simulink model "sf_mask_basic"  (R2017b)
settings: Solver=VariableStepDiscrete  StartTime=0.0  StopTime=300.0  MaxStep=2.0  RelTol=1e-3  EnableMultiTasking=on
libraries: sf_mask_lib x1
settings Model: Creator=The MathWorks, Inc.  LastModifiedBy=The MathWorks, Inc.
settings DataIOCC: LimitDataPoints=on  SaveFormat=Array
settings OptimizationCC: ExpressionDepthLimit=2147483647  LifeSpan=inf
settings DebuggingCC: UnderspecifiedInitializationDetection=Classic  MergeDetectMultiDrivingBlocksExec=none  SolverPrmCheckMsg=warning  StateNameClashWarn=warning  SFUnexpectedBacktrackingDiag=warning  SFNoUnconditionalDefaultTransitionDiag=warning  SFExecutionAtInitializationDiag=none
settings HardwareCC: ProdBitPerPointer=32  ProdBitPerSizeT=32  ProdBitPerPtrDiffT=32  ProdLargestAtomicFloat=None  ProdIntDivRoundTo=Undefined  ProdEndianess=Unspecified  ProdWordSize=32  ProdHWDeviceType=32-bit Generic
settings ModelReferenceCC: PropagateSignalLabelsOutOfModel=off
settings CodeAppCC: StateflowObjectComments=on
settings GRTTargetCC: TargetLangStandard=C89/C90 (ANSI)  GeneratePreprocessorConditionals=Disable all
settings ConfigComp: CovMetricSettings=dw  CovHtmlReporting=on  CovSaveCumulativeToWorkspaceVar=on  CovSaveSingleToWorkspaceVar=on  CovExternalEMLEnable=off

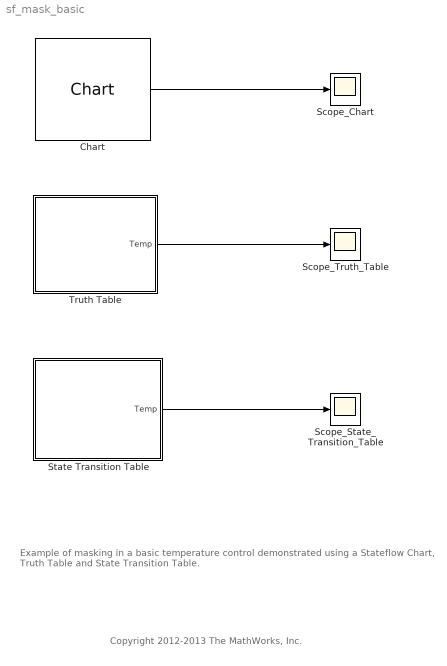
== system sf_mask_basic ==
  note: Copyright 2012-2013 The MathWorks, Inc.
  note: Example of masking in a basic temperature control demonstrated using a
      |  Stateflow Chart, Truth Table and State Transition Table.
  Chart : sf_mask_lib/Chart  AmbTemp=85  DesiredTemp=70  btuSetting=20000 BTUs
      settings: SourceProductName=Stateflow  SourceProductBaseCode=SF
  Scope_Chart : Scope
  Scope_State_Transition_Table : Scope
  Scope_Truth_Table : Scope
  State Transition Table : State Transition Table  TreatAsAtomicUnit=on  mask{AmbTemp=85, DesiredTemp=70, btuSetting=20000 BTU}
      mask prompts: AmbTemp "Ambient Temperature"; DesiredTemp "Desired Temperature"; btuSetting "AC Power"
      mask init:
      | if btuSetting == 1
      |     btuValue = 10000;
      | elseif btuSetting == 2
      |     btuValue = 20000;
      | end
  Truth Table : Truth Table  TreatAsAtomicUnit=on  mask{AmbTemp=85, DesiredTemp=70, btuSetting=20000 BTU}
      mask prompts: AmbTemp "Ambient Temperature"; DesiredTemp "Desired Temperature"; btuSetting "AC Power"
      mask init:
      | if btuSetting == 1
      |     btuValue = 10000;
      | elseif btuSetting == 2
      |     btuValue = 20000;
      | end
  wires:
  Chart/1 -> Scope_Chart/1
  Truth Table/1(Temp) -> Scope_Truth_Table/1
  State Transition Table/1(Temp) -> Scope_State_Transition_Table/1

== matlab function sf_mask_basic/Truth Table ==
  data: Temp output; AmbTemp parameter double; DesiredTemp parameter double; TempStore local double =AmbTemp; btuValue parameter double
function Temp = fcn(AmbTemp, DesiredTemp, btuValue)

INIT();

aVarTruthTableCondition_1 = false;


% Temperature is Less than Desired

aVarTruthTableCondition_1 = logical(TempStore < DesiredTemp);

if (aVarTruthTableCondition_1)
    AC_OFF();
else % Default
    AC_ON();
end

function INIT()


Temp = TempStore;

function AC_ON()

% AC is ON

TempStore = Temp - btuValue/20000;

function AC_OFF()

% AC is OFF

TempStore = Temp + 0.05*(AmbTemp - Temp);

== stateflow chart sf_mask_basic/State Transition Table ==
  state AC_OFF
    entry,during:Temp = Temp + 0.05*(AmbTemp - Temp);
  state AC_ON
    entry,during:Temp = Temp - btuValue/20000;
  (default) -> AC_OFF : {Temp = AmbTemp;}
  AC_OFF -> AC_ON : [Temp >= DesiredTemp]
  AC_ON -> AC_OFF : [Temp < DesiredTemp]
  data: Temp output; DesiredTemp parameter; AmbTemp parameter; btuValue parameter
